simulink model "RaceCar_7DOF_ActiveSuspension"  (R2026a)
settings: Solver=ode4  StopTime=5  FixedStep=0.001
undefined symbols (not defined in the file): a, active_mode, b, bump_duration, bump_height, c_sf, C_sky, c_sr, controller_mode, F_act_max, Ixx, Iyy, K_lqr, k_sf, k_sr, k_t, kerb_duration, kerb_height, m_s, m_uf, m_ur, phi0, phi_dot0, sweep_amplitude, sweep_time, t_bump_front, t_bump_rear, t_f, t_kerb_front, t_kerb_rear, t_r, theta0, theta_dot0, z_s0, z_s_dot0, z_u_FL0, z_u_FL_dot0, z_u_FR0, z_u_FR_dot0, z_u_RL0, z_u_RL_dot0, z_u_RR0, z_u_RR_dot0
libraries: simulink x1
settings Model: Creator=chami  LastModifiedBy=chami

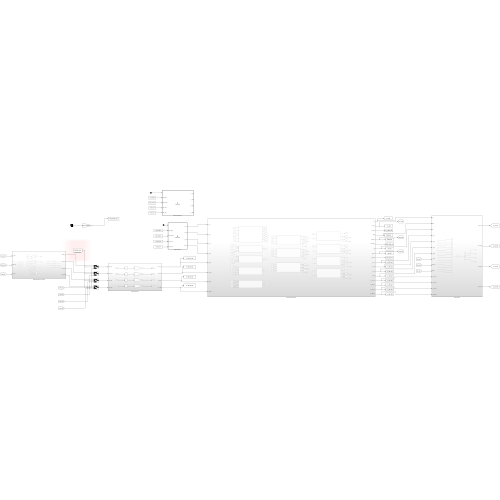
[thumbnail: Simulink's stored preview of the top-level diagram]
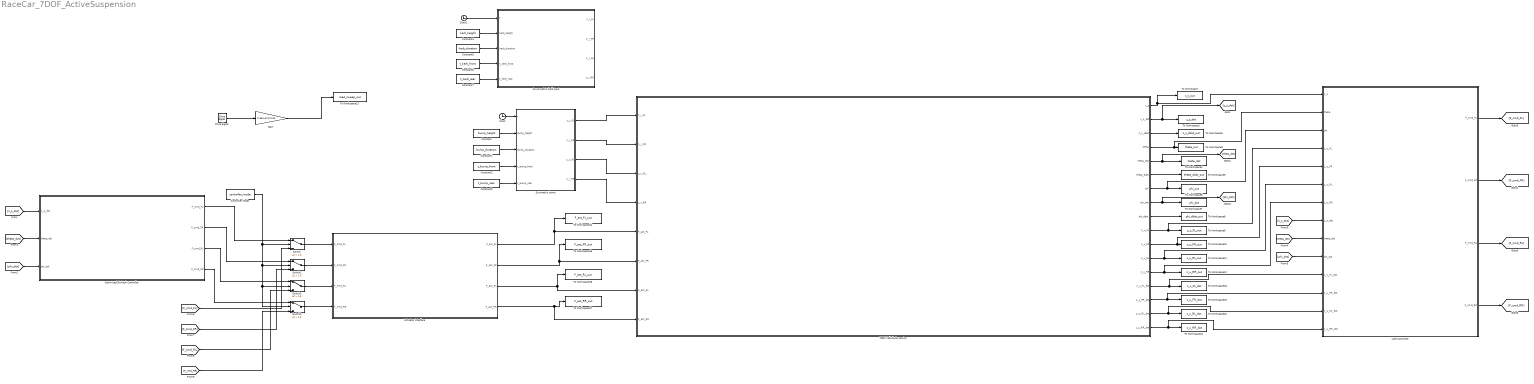
== system RaceCar_7DOF_ActiveSuspension ==
  7DOF Vehicle Dynamics : Subsystem
  Actuator Interface : Subsystem
  Asymmetric Kerb Input : MATLAB Function  TreatAsAtomicUnit=on
  Chirp Signal : simulink/Sources/Chirp Signal  f1=sweep_f_start  T=sweep_time  f2=sweep_f_end
  Clock : Clock
  Clock1 : Clock
  Constant : Constant  Value=bump_height
  Constant1 : Constant  Value=bump_duration
  Constant2 : Constant  Value=t_bump_front
  Constant3 : Constant  Value=t_bump_rear
  Constant4 : Constant  Value=kerb_height
  Constant5 : Constant  Value=kerb_duration
  Constant6 : Constant  Value=t_kerb_front
  Constant7 : Constant  Value=t_kerb_rear
  Controller Mode : Constant  Value=controller_mode
  Gain : Gain  Gain=sweep_amplitude
  LQR Controller : Subsystem
  Optimized Skyhook Controller : Subsystem
  Switch{,1..3} (4 alike) : Switch  Criteria=u2 > Threshold  Threshold=1.5  SaturateOnIntegerOverflow=off  InputSameDT=off
  Symmetric bump : MATLAB Function  TreatAsAtomicUnit=on
  To Workspace : ToWorkspace  VariableName=z_s_out  SaveFormat=Timeseries  SampleTime=-1
  To Workspace1 : ToWorkspace  VariableName=z_s_dot  SaveFormat=Timeseries  SampleTime=-1
  To Workspace10 : ToWorkspace  VariableName=z_u_FR_out  SaveFormat=Timeseries  SampleTime=-1
  To Workspace11 : ToWorkspace  VariableName=z_u_RL_out  SaveFormat=Timeseries  SampleTime=-1
  To Workspace12 : ToWorkspace  VariableName=z_u_RR_out  SaveFormat=Timeseries  SampleTime=-1
  To Workspace13 : ToWorkspace  VariableName=road_sweep_out  SaveFormat=Timeseries  SampleTime=-1
  To Workspace14 : ToWorkspace  VariableName=F_act_FL_out  SaveFormat=Timeseries  SampleTime=-1
  To Workspace15 : ToWorkspace  VariableName=F_act_FR_out  SaveFormat=Timeseries  SampleTime=-1
  To Workspace16 : ToWorkspace  VariableName=F_act_RL_out  SaveFormat=Timeseries  SampleTime=-1
  To Workspace17 : ToWorkspace  VariableName=F_act_RR_out  SaveFormat=Timeseries  SampleTime=-1
  To Workspace18 : ToWorkspace  VariableName=z_u_FL_dot  SaveFormat=Timeseries  SampleTime=-1
  To Workspace19 : ToWorkspace  VariableName=z_u_FR_dot  SaveFormat=Timeseries  SampleTime=-1
  To Workspace2 : ToWorkspace  VariableName=z_s_ddot_out  SaveFormat=Timeseries  SampleTime=-1
  To Workspace20 : ToWorkspace  VariableName=z_u_RL_dot  SaveFormat=Timeseries  SampleTime=-1
  To Workspace21 : ToWorkspace  VariableName=z_u_RR_dot  SaveFormat=Timeseries  SampleTime=-1
  To Workspace3 : ToWorkspace  VariableName=theta_out  SaveFormat=Timeseries  SampleTime=-1
  To Workspace4 : ToWorkspace  VariableName=theta_dot  SaveFormat=Timeseries  SampleTime=-1
  To Workspace5 : ToWorkspace  VariableName=theta_ddot_out  SaveFormat=Timeseries  SampleTime=-1
  To Workspace6 : ToWorkspace  VariableName=phi_out  SaveFormat=Timeseries  SampleTime=-1
  To Workspace7 : ToWorkspace  VariableName=phi_dot  SaveFormat=Timeseries  SampleTime=-1
  To Workspace8 : ToWorkspace  VariableName=phi_ddot_out  SaveFormat=Timeseries  SampleTime=-1
  To Workspace9 : ToWorkspace  VariableName=z_u_FL_out  SaveFormat=Timeseries  SampleTime=-1
  wires:
  7DOF Vehicle Dynamics/1(z_s) -> To Workspace/1, LQR Controller/1(z_s)
  7DOF Vehicle Dynamics/2(z_s_dot) -> [z_s_dot], To Workspace1/1
  7DOF Vehicle Dynamics/3(z_s_ddot) -> To Workspace2/1
  7DOF Vehicle Dynamics/6(theta_ddot) -> To Workspace5/1
  7DOF Vehicle Dynamics/5(theta_dot) -> To Workspace4/1, [theta_dot]
  7DOF Vehicle Dynamics/4(theta) -> LQR Controller/2(theta), To Workspace3/1
  7DOF Vehicle Dynamics/8(phi_dot) -> [phi_dot], To Workspace7/1
  7DOF Vehicle Dynamics/7(phi) -> LQR Controller/3(phi), To Workspace6/1
  7DOF Vehicle Dynamics/9(phi_ddot) -> To Workspace8/1
  7DOF Vehicle Dynamics/10(z_u_FL) -> LQR Controller/4(z_u_FL), To Workspace9/1
  7DOF Vehicle Dynamics/11(z_u_FR) -> LQR Controller/5(z_u_FR), To Workspace10/1
  7DOF Vehicle Dynamics/12(z_u_RL) -> LQR Controller/6(z_u_RL), To Workspace11/1
  7DOF Vehicle Dynamics/13(z_u_RR) -> LQR Controller/7(z_u_RR), To Workspace12/1
  Clock/1 -> Symmetric bump/1(t)
  Constant/1 -> Symmetric bump/2(bump_height)
  Constant1/1 -> Symmetric bump/3(bump_duration)
  Constant2/1 -> Symmetric bump/4(t_bump_front)
  Constant3/1 -> Symmetric bump/5(t_bump_rear)
  Chirp Signal/1 -> Gain/1
  Gain/1 -> To Workspace13/1
  Actuator Interface/1(F_act_FL) -> To Workspace14/1, 7DOF Vehicle Dynamics/5(F_act_FL)
  Actuator Interface/2(F_act_FR) -> To Workspace15/1, 7DOF Vehicle Dynamics/6(F_act_FR)
  Actuator Interface/3(F_act_RL) -> To Workspace16/1, 7DOF Vehicle Dynamics/7(F_act_RL)
  Actuator Interface/4(F_act_RR) -> To Workspace17/1, 7DOF Vehicle Dynamics/8(F_act_RR)
  [z_s_dot] -> Optimized Skyhook Controller/1(z_s_dot)
  [theta_dot] -> Optimized Skyhook Controller/2(theta_dot)
  [phi_dot] -> Optimized Skyhook Controller/3(phi_dot)
  Clock1/1 -> Asymmetric Kerb Input/1(t)
  Constant4/1 -> Asymmetric Kerb Input/2(kerb_height)
  Constant5/1 -> Asymmetric Kerb Input/3(kerb_duration)
  Constant6/1 -> Asymmetric Kerb Input/4(t_kerb_front)
  Constant7/1 -> Asymmetric Kerb Input/5(t_kerb_rear)
  7DOF Vehicle Dynamics/14(z_u_FL_dot) -> LQR Controller/11(z_u_FL_dot), To Workspace18/1
  7DOF Vehicle Dynamics/15(z_u_FR_dot) -> LQR Controller/12(z_u_FR_dot), To Workspace19/1
  7DOF Vehicle Dynamics/16(z_u_RL_dot) -> LQR Controller/13(z_u_RL_dot), To Workspace20/1
  7DOF Vehicle Dynamics/17(z_u_RR_dot) -> LQR Controller/14(z_u_RR_dot), To Workspace21/1
  [phi_dot] -> LQR Controller/10(phi_dot)
  [theta_dot] -> LQR Controller/9(theta_dot)
  [z_s_dot] -> LQR Controller/8(z_s_dot)
  LQR Controller/1(F_cmd_FL) -> [F_cmd_FL]
  LQR Controller/2(F_cmd_FR) -> [F_cmd_FR]
  LQR Controller/3(F_cmd_RL) -> [F_cmd_RL]
  LQR Controller/4(F_cmd_RR) -> [F_cmd_RR]
  Symmetric bump/1(z_r_FL) -> 7DOF Vehicle Dynamics/1(z_r_FL)
  Symmetric bump/2(z_r_FR) -> 7DOF Vehicle Dynamics/2(z_r_FR)
  Symmetric bump/3(z_r_RL) -> 7DOF Vehicle Dynamics/3(z_r_RL)
  Symmetric bump/4(z_r_RR) -> 7DOF Vehicle Dynamics/4(z_r_RR)
  Switch/1 -> Actuator Interface/1("F_cmd_FL ")
  Switch1/1 -> Actuator Interface/2(F_cmd_FR)
  Switch2/1 -> Actuator Interface/3(F_cmd_RL)
  Switch3/1 -> Actuator Interface/4(F_cmd_RR)
  Optimized Skyhook Controller/1(F_cmd_FL) -> Switch/1
  Optimized Skyhook Controller/2(F_cmd_FR) -> Switch1/1
  Optimized Skyhook Controller/3(F_cmd_RL) -> Switch2/1
  Optimized Skyhook Controller/4(F_cmd_RR) -> Switch3/1
  [F_cmd_FL] -> Switch/3
  [F_cmd_FR] -> Switch1/3
  [F_cmd_RL] -> Switch2/3
  [F_cmd_RR] -> Switch3/3
  Controller Mode/1 -> Switch/2, Switch1/2, Switch2/2, Switch3/2

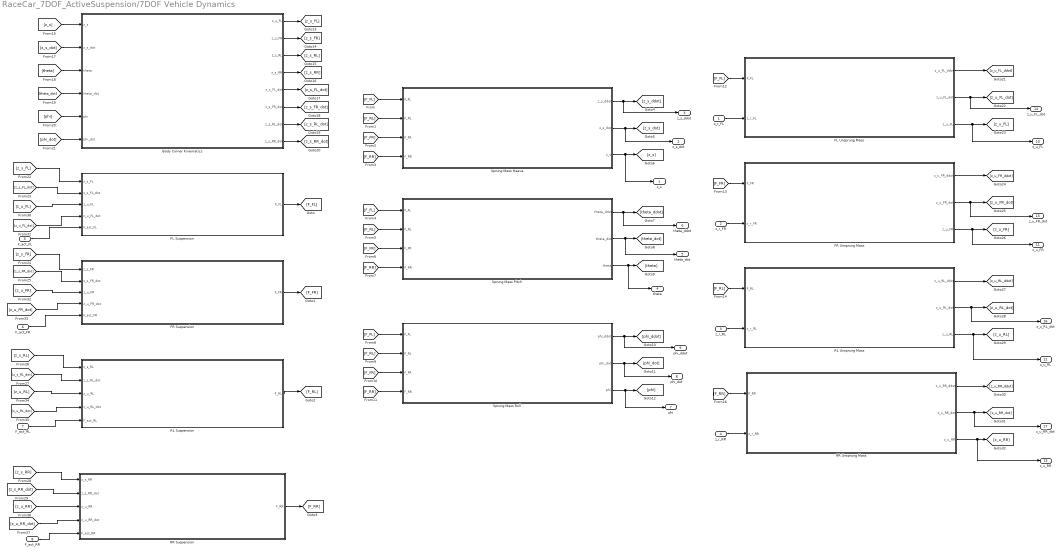
== system RaceCar_7DOF_ActiveSuspension/7DOF Vehicle Dynamics ==
  z_r_FL : Inport
  z_r_FR : Inport  Port=2
  z_r_RL : Inport  Port=3
  z_r_RR : Inport  Port=4
  F_act_FL : Inport  Port=5
  F_act_FR : Inport  Port=6
  F_act_RL : Inport  Port=7
  F_act_RR : Inport  Port=8
  Body Corner Kinematics : Subsystem
  "FL Suspension " : Subsystem
  FL Unsprung Mass : Subsystem
  FR Suspension : Subsystem
  FR Unsprung Mass : Subsystem
  RL Suspension : Subsystem
  RL Unsprung Mass : Subsystem
  RR Suspension : Subsystem
  RR Unsprung Mass : Subsystem
  Sprung Mass Heave : Subsystem
  Sprung Mass Pitch : Subsystem
  Sprung Mass Roll : Subsystem
  z_s : Outport
  z_s_dot : Outport  Port=2
  z_s_ddot : Outport  Port=3
  theta : Outport  Port=4
  theta_dot : Outport  Port=5
  theta_ddot : Outport  Port=6
  phi : Outport  Port=7
  phi_dot : Outport  Port=8
  phi_ddot : Outport  Port=9
  z_u_FL : Outport  Port=10
  z_u_FR : Outport  Port=11
  z_u_RL : Outport  Port=12
  z_u_RR : Outport  Port=13
  z_u_FL_dot : Outport  Port=14
  z_u_FR_dot : Outport  Port=15
  z_u_RL_dot : Outport  Port=16
  z_u_RR_dot : Outport  Port=17
  wires:
  [F_FL] -> Sprung Mass Pitch/1(F_FL)
  Body Corner Kinematics/2(z_s_FR) -> [z_s_FR]
  [z_u_FL_dot] -> "FL Suspension "/4(z_u_FL_dot)
  [phi] -> Body Corner Kinematics/5(phi)
  Sprung Mass Roll/3(phi) -> phi/1, [phi]
  [z_u_RL_dot] -> RL Suspension/4(z_u_RL_dot)
  [F_FR] -> Sprung Mass Roll/3(F_FR)
  [z_s_RL] -> RL Suspension/1(z_s_RL)
  FL Unsprung Mass/2(z_u_FL_dot) -> z_u_FL_dot/1, [z_u_FL_dot]
  [z_s] -> Body Corner Kinematics/1(z_s)
  [theta] -> Body Corner Kinematics/3(theta)
  [z_s_FL] -> "FL Suspension "/1(z_s_FL)
  FR Unsprung Mass/3(z_u_FR) -> z_u_FR/1, [z_u_FR]
  [z_s_RR_dot] -> RR Suspension/2(z_s_RR_dot)
  FL Unsprung Mass/1(z_u_FL_ddot) -> [z_u_FL_ddot]
  Sprung Mass Pitch/1(theta_ddot) -> theta_ddot/1, [theta_ddot]
  Sprung Mass Pitch/3(theta) -> theta/1, [theta]
  [F_RL] -> Sprung Mass Heave/2(F_RL)
  Body Corner Kinematics/1(z_s_FL) -> [z_s_FL]
  [z_s_FR] -> FR Suspension/1(z_s_FR)
  Body Corner Kinematics/4(z_s_RR) -> [z_s_RR]
  [z_u_RR_dot] -> RR Suspension/4(z_u_RR_dot)
  FR Suspension/1(F_FR) -> [F_FR]
  FR Unsprung Mass/1(z_u_FR_ddot) -> [z_u_FR_ddot]
  RL Unsprung Mass/1(z_u_RL_ddot) -> [z_u_RL_ddot]
  [F_FR] -> Sprung Mass Pitch/3(F_FR)
  [F_RL] -> RL Unsprung Mass/1(F_RL)
  Body Corner Kinematics/6(z_s_FR_dot) -> [z_s_FR_dot]
  [z_s_dot] -> Body Corner Kinematics/2(z_s_dot)
  [z_u_FR] -> FR Suspension/3(z_u_FR)
  [z_s_FR_dot] -> FR Suspension/2(z_s_FR_dot)
  RR Suspension/1(F_RR) -> [F_RR]
  Sprung Mass Heave/2(z_s_dot) -> z_s_dot/1, [z_s_dot]
  Sprung Mass Roll/2(phi_dot) -> phi_dot/1, [phi_dot]
  Body Corner Kinematics/5(z_s_FL_dot) -> [z_s_FL_dot]
  [z_u_FL] -> "FL Suspension "/3(z_u_FL)
  [z_u_RL] -> RL Suspension/3(z_u_RL)
  Sprung Mass Heave/1(z_s_ddot) -> z_s_ddot/1, [z_s_ddot]
  [z_s_RR] -> RR Suspension/1(z_s_RR)
  [F_RR] -> Sprung Mass Heave/4(F_RR)
  [F_FL] -> FL Unsprung Mass/1(F_FL)
  [theta_dot] -> Body Corner Kinematics/4(theta_dot)
  [F_FL] -> Sprung Mass Heave/1(F_FL)
  [F_FL] -> Sprung Mass Roll/1(F_FL)
  [z_s_FL_dot] -> "FL Suspension "/2(z_s_FL_dot)
  Body Corner Kinematics/8(z_s_RR_dot) -> [z_s_RR_dot]
  [F_RR] -> RR Unsprung Mass/1(F_RR)
  [z_u_FR_dot] -> FR Suspension/4(z_u_FR_dot)
  [z_u_RR] -> RR Suspension/3(z_u_RR)
  [F_RL] -> Sprung Mass Pitch/2(F_RL)
  Sprung Mass Heave/3(z_s) -> z_s/1, [z_s]
  RL Suspension/1(F_RL) -> [F_RL]
  RR Unsprung Mass/3(z_u_RR) -> z_u_RR/1, [z_u_RR]
  FL Unsprung Mass/3(z_u_FL) -> z_u_FL/1, [z_u_FL]
  RL Unsprung Mass/3(z_u_RL) -> z_u_RL/1, [z_u_RL]
  FR Unsprung Mass/2(z_u_FR_dot) -> z_u_FR_dot/1, [z_u_FR_dot]
  [F_FR] -> FR Unsprung Mass/1(F_FR)
  "FL Suspension "/1(F_FL) -> [F_FL]
  [F_RR] -> Sprung Mass Roll/4(F_RR)
  Sprung Mass Roll/1(phi_ddot) -> phi_ddot/1, [phi_ddot]
  RR Unsprung Mass/1(z_u_RR_ddot) -> [z_u_RR_ddot]
  [F_RR] -> Sprung Mass Pitch/4(F_RR)
  RR Unsprung Mass/2(z_u_RR_dot) -> z_u_RR_dot/1, [z_u_RR_dot]
  [F_RL] -> Sprung Mass Roll/2(F_RL)
  Sprung Mass Pitch/2(theta_dot) -> theta_dot/1, [theta_dot]
  [F_FR] -> Sprung Mass Heave/3(F_FR)
  [z_s_RL_dot] -> RL Suspension/2(z_s_RL_dot)
  [phi_dot] -> Body Corner Kinematics/6(phi_dot)
  Body Corner Kinematics/7(z_s_RL_dot) -> [z_s_RL_dot]
  RL Unsprung Mass/2(z_u_RL_dot) -> z_u_RL_dot/1, [z_u_RL_dot]
  Body Corner Kinematics/3(z_s_RL) -> [z_s_RL]
  z_r_FL/1 -> FL Unsprung Mass/2(z_r_FL)
  z_r_FR/1 -> FR Unsprung Mass/2(z_r_FR)
  z_r_RL/1 -> RL Unsprung Mass/2(z_r_RL)
  z_r_RR/1 -> RR Unsprung Mass/2(z_r_RR)
  F_act_FL/1 -> "FL Suspension "/5(F_act_FL)
  F_act_FR/1 -> FR Suspension/5(F_act_FR)
  F_act_RL/1 -> RL Suspension/5(F_act_RL)
  F_act_RR/1 -> RR Suspension/5(F_act_RR)

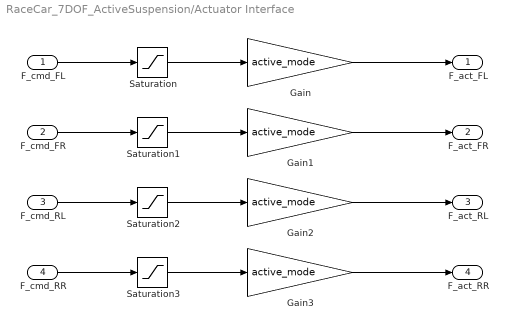
== system RaceCar_7DOF_ActiveSuspension/Actuator Interface ==
  "F_cmd_FL " : Inport
  F_cmd_FR : Inport  Port=2
  F_cmd_RL : Inport  Port=3
  F_cmd_RR : Inport  Port=4
  Gain{,1..3} (4 alike) : Gain  Gain=active_mode
  Saturation{,1..3} (4 alike) : Saturate  UpperLimit=F_act_max  LowerLimit=-F_act_max
  F_act_FL : Outport
  F_act_FR : Outport  Port=2
  F_act_RL : Outport  Port=3
  F_act_RR : Outport  Port=4
  wires:
  Saturation/1 -> Gain/1
  Saturation1/1 -> Gain1/1
  Saturation2/1 -> Gain2/1
  Saturation3/1 -> Gain3/1
  "F_cmd_FL "/1 -> Saturation/1
  F_cmd_FR/1 -> Saturation1/1
  F_cmd_RL/1 -> Saturation2/1
  F_cmd_RR/1 -> Saturation3/1
  Gain/1 -> F_act_FL/1
  Gain1/1 -> F_act_FR/1
  Gain2/1 -> F_act_RL/1
  Gain3/1 -> F_act_RR/1

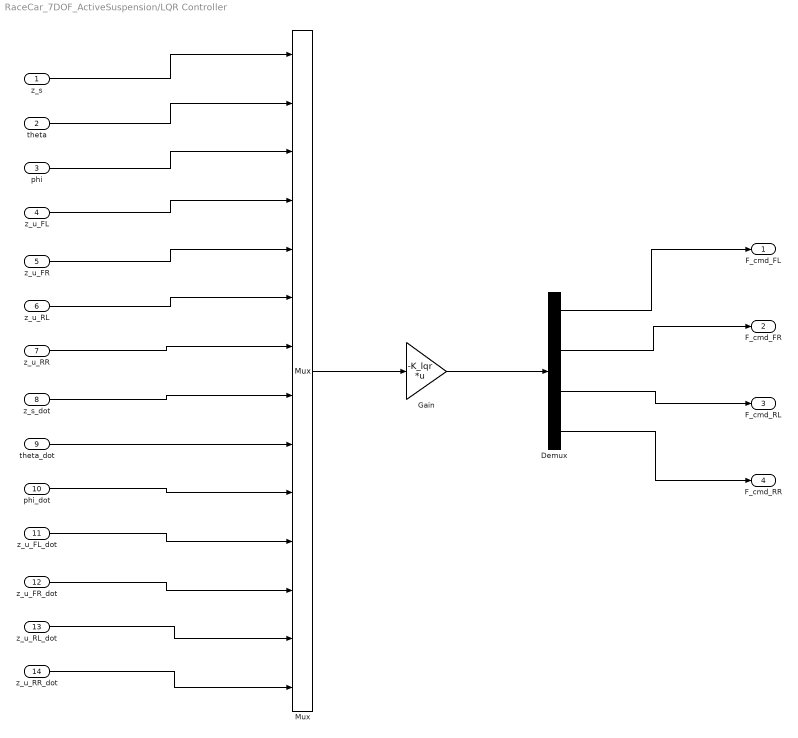
== system RaceCar_7DOF_ActiveSuspension/LQR Controller ==
  z_s : Inport
  theta : Inport  Port=2
  phi : Inport  Port=3
  z_u_FL : Inport  Port=4
  z_u_FR : Inport  Port=5
  z_u_RL : Inport  Port=6
  z_u_RR : Inport  Port=7
  z_s_dot : Inport  Port=8
  theta_dot : Inport  Port=9
  phi_dot : Inport  Port=10
  z_u_FL_dot : Inport  Port=11
  z_u_FR_dot : Inport  Port=12
  z_u_RL_dot : Inport  Port=13
  z_u_RR_dot : Inport  Port=14
  Demux : Demux
  Gain : Gain  Gain=-K_lqr  Multiplication=Matrix(K*u)
  Mux : Mux  Inputs=14
  F_cmd_FL : Outport
  F_cmd_FR : Outport  Port=2
  F_cmd_RL : Outport  Port=3
  F_cmd_RR : Outport  Port=4
  wires:
  z_s/1 -> Mux/1
  theta/1 -> Mux/2
  phi/1 -> Mux/3
  z_u_FL/1 -> Mux/4
  z_u_FR/1 -> Mux/5
  z_u_RL/1 -> Mux/6
  z_u_RR/1 -> Mux/7
  z_s_dot/1 -> Mux/8
  theta_dot/1 -> Mux/9
  phi_dot/1 -> Mux/10
  z_u_FL_dot/1 -> Mux/11
  z_u_FR_dot/1 -> Mux/12
  z_u_RL_dot/1 -> Mux/13
  z_u_RR_dot/1 -> Mux/14
  Mux/1 -> Gain/1
  Gain/1 -> Demux/1
  Demux/1 -> F_cmd_FL/1
  Demux/2 -> F_cmd_FR/1
  Demux/3 -> F_cmd_RL/1
  Demux/4 -> F_cmd_RR/1

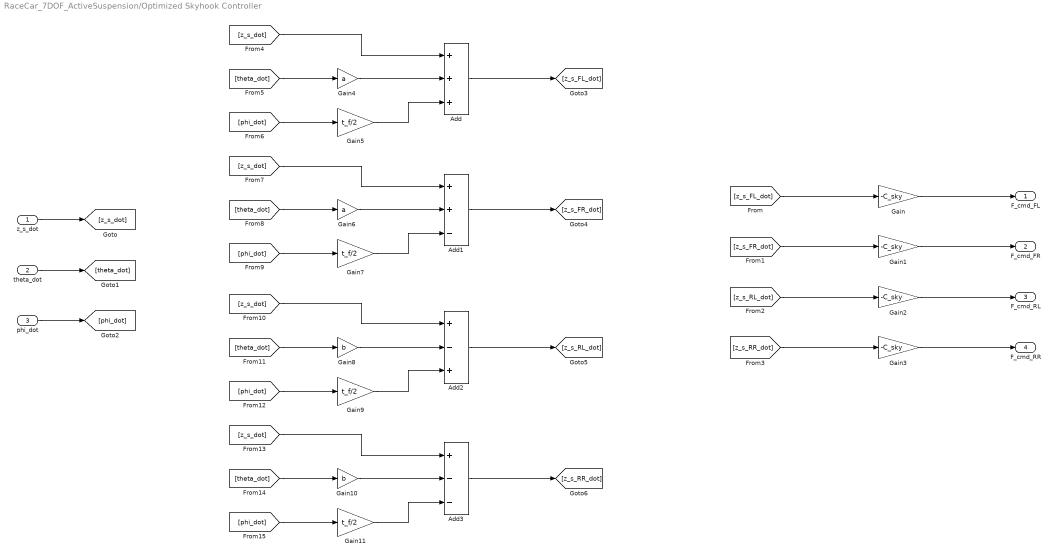
== system RaceCar_7DOF_ActiveSuspension/Optimized Skyhook Controller ==
  z_s_dot : Inport
  theta_dot : Inport  Port=2
  phi_dot : Inport  Port=3
  Add : Sum  Inputs=+++
  Add1 : Sum  Inputs=++-
  Add2 : Sum  Inputs=+-+
  Add3 : Sum  Inputs=+--
  Gain{,1..3} (4 alike) : Gain  Gain=-C_sky
  Gain10 : Gain  Gain=b
  Gain{5,7,9,11} (4 alike) : Gain  Gain=t_f/2
  Gain4 : Gain  Gain=a
  Gain6 : Gain  Gain=a
  Gain8 : Gain  Gain=b
  F_cmd_FL : Outport
  F_cmd_FR : Outport  Port=2
  F_cmd_RL : Outport  Port=3
  F_cmd_RR : Outport  Port=4
  wires:
  [z_s_FL_dot] -> Gain/1
  [z_s_FR_dot] -> Gain1/1
  [z_s_RL_dot] -> Gain2/1
  [z_s_RR_dot] -> Gain3/1
  Gain/1 -> F_cmd_FL/1
  Gain1/1 -> F_cmd_FR/1
  Gain2/1 -> F_cmd_RL/1
  Gain3/1 -> F_cmd_RR/1
  z_s_dot/1 -> [z_s_dot]
  theta_dot/1 -> [theta_dot]
  phi_dot/1 -> [phi_dot]
  [theta_dot] -> Gain4/1
  [phi_dot] -> Gain5/1
  Gain4/1 -> Add/2
  [z_s_dot] -> Add/1
  Gain5/1 -> Add/3
  Add/1 -> [z_s_FL_dot]
  Add1/1 -> [z_s_FR_dot]
  Gain7/1 -> Add1/3
  [z_s_dot] -> Add1/1
  Gain6/1 -> Add1/2
  [phi_dot] -> Gain7/1
  [theta_dot] -> Gain6/1
  [theta_dot] -> Gain10/1
  [phi_dot] -> Gain11/1
  Gain10/1 -> Add3/2
  [z_s_dot] -> Add3/1
  Gain11/1 -> Add3/3
  Add3/1 -> [z_s_RR_dot]
  Add2/1 -> [z_s_RL_dot]
  Gain9/1 -> Add2/3
  [z_s_dot] -> Add2/1
  Gain8/1 -> Add2/2
  [phi_dot] -> Gain9/1
  [theta_dot] -> Gain8/1

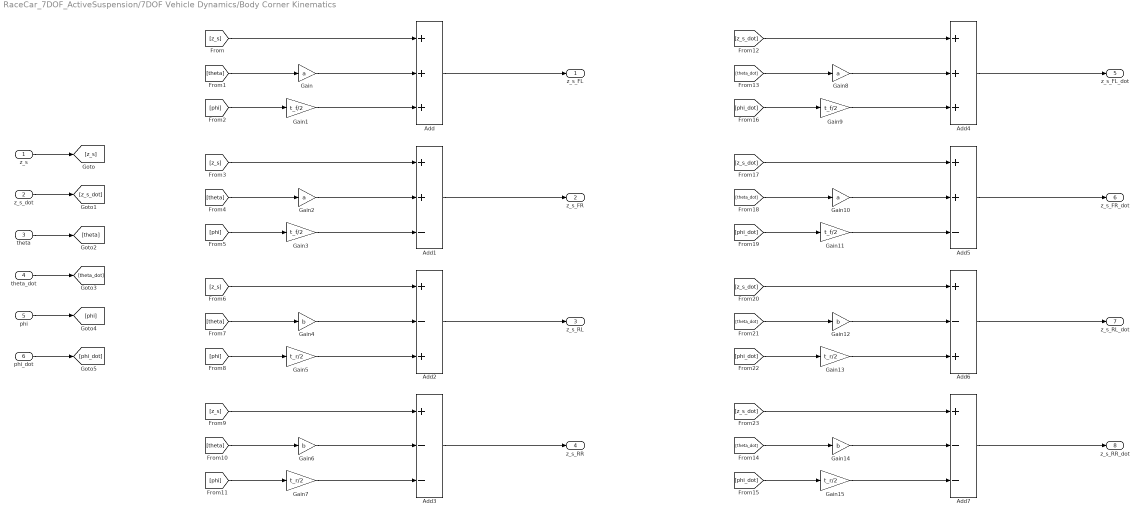
== system RaceCar_7DOF_ActiveSuspension/7DOF Vehicle Dynamics/Body Corner Kinematics ==
  z_s : Inport
  z_s_dot : Inport  Port=2
  theta : Inport  Port=3
  theta_dot : Inport  Port=4
  phi : Inport  Port=5
  phi_dot : Inport  Port=6
  Add : Sum  Inputs=+++
  Add1 : Sum  Inputs=++-
  Add2 : Sum  Inputs=+-+
  Add3 : Sum  Inputs=+--
  Add4 : Sum  Inputs=+++
  Add5 : Sum  Inputs=++-
  Add6 : Sum  Inputs=+-+
  Add7 : Sum  Inputs=+--
  Gain{,2,8,10} (4 alike) : Gain  Gain=a
  Gain{1,3,9,11} (4 alike) : Gain  Gain=t_f/2
  Gain{4,6,12,14} (4 alike) : Gain  Gain=b
  Gain{5,7,13,15} (4 alike) : Gain  Gain=t_r/2
  z_s_FL : Outport
  z_s_FR : Outport  Port=2
  z_s_RL : Outport  Port=3
  z_s_RR : Outport  Port=4
  z_s_FL_dot : Outport  Port=5
  z_s_FR_dot : Outport  Port=6
  z_s_RL_dot : Outport  Port=7
  z_s_RR_dot : Outport  Port=8
  wires:
  Gain/1 -> Add/2
  Gain1/1 -> Add/3
  Add/1 -> z_s_FL/1
  z_s/1 -> [z_s]
  z_s_dot/1 -> [z_s_dot]
  theta/1 -> [theta]
  theta_dot/1 -> [theta_dot]
  phi/1 -> [phi]
  phi_dot/1 -> [phi_dot]
  [z_s] -> Add/1
  [theta] -> Gain/1
  [phi] -> Gain1/1
  [phi] -> Gain3/1
  [theta] -> Gain2/1
  [z_s] -> Add1/1
  Add1/1 -> z_s_FR/1
  Gain3/1 -> Add1/3
  Gain2/1 -> Add1/2
  [phi] -> Gain5/1
  [theta] -> Gain4/1
  [z_s] -> Add2/1
  Add2/1 -> z_s_RL/1
  Gain5/1 -> Add2/3
  Gain4/1 -> Add2/2
  Gain6/1 -> Add3/2
  Gain7/1 -> Add3/3
  Add3/1 -> z_s_RR/1
  [z_s] -> Add3/1
  [theta] -> Gain6/1
  [phi] -> Gain7/1
  [phi_dot] -> Gain15/1
  [theta_dot] -> Gain14/1
  [z_s_dot] -> Add7/1
  Add7/1 -> z_s_RR_dot/1
  Gain15/1 -> Add7/3
  Gain14/1 -> Add7/2
  Gain12/1 -> Add6/2
  Gain13/1 -> Add6/3
  Add6/1 -> z_s_RL_dot/1
  [z_s_dot] -> Add6/1
  [theta_dot] -> Gain12/1
  [phi_dot] -> Gain13/1
  Gain10/1 -> Add5/2
  Gain11/1 -> Add5/3
  Add5/1 -> z_s_FR_dot/1
  [z_s_dot] -> Add5/1
  [theta_dot] -> Gain10/1
  [phi_dot] -> Gain11/1
  [phi_dot] -> Gain9/1
  [theta_dot] -> Gain8/1
  [z_s_dot] -> Add4/1
  Add4/1 -> z_s_FL_dot/1
  Gain9/1 -> Add4/3
  Gain8/1 -> Add4/2

== system RaceCar_7DOF_ActiveSuspension/7DOF Vehicle Dynamics/FL Suspension  ==
  z_s_FL : Inport
  z_s_FL_dot : Inport  Port=2
  z_u_FL : Inport  Port=3
  z_u_FL_dot : Inport  Port=4
  F_act_FL : Inport  Port=5
  Add : Sum  Inputs=+-
  Add1 : Sum  Inputs=+-
  Add2 : Sum  Inputs=+++
  Gain : Gain  Gain=-k_sf
  Gain1 : Gain  Gain=-c_sf
  F_FL : Outport
  wires:
  z_u_FL/1 -> Add/2
  z_s_FL/1 -> Add/1
  z_u_FL_dot/1 -> Add1/2
  z_s_FL_dot/1 -> Add1/1
  Add/1 -> Gain/1  "delta_FL"
  Add1/1 -> Gain1/1  "delta_FL_dot"
  Add2/1 -> F_FL/1
  Gain/1 -> Add2/1  "Fs_FL"
  Gain1/1 -> Add2/2  "Fd_FL"
  F_act_FL/1 -> Add2/3

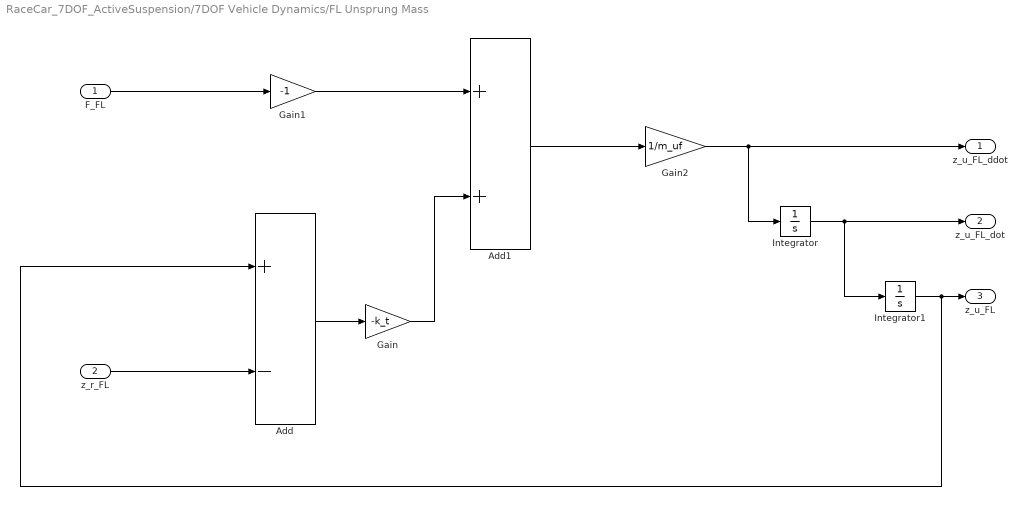
== system RaceCar_7DOF_ActiveSuspension/7DOF Vehicle Dynamics/FL Unsprung Mass ==
  F_FL : Inport
  z_r_FL : Inport  Port=2
  Add : Sum  Inputs=+-
  Add1 : Sum
  Gain : Gain  Gain=-k_t
  Gain1 : Gain  Gain=-1
  Gain2 : Gain  Gain=1/m_uf
  Integrator : Integrator  InitialCondition=z_u_FL_dot0
  Integrator1 : Integrator  InitialCondition=z_u_FL0
  z_u_FL_ddot : Outport
  z_u_FL_dot : Outport  Port=2
  z_u_FL : Outport  Port=3
  wires:
  Integrator1/1 -> Add/1, z_u_FL/1
  Integrator/1 -> z_u_FL_dot/1, Integrator1/1
  z_r_FL/1 -> Add/2
  Add/1 -> Gain/1
  Gain/1 -> Add1/2
  F_FL/1 -> Gain1/1
  Gain1/1 -> Add1/1
  Add1/1 -> Gain2/1
  Gain2/1 -> Integrator/1, z_u_FL_ddot/1

== system RaceCar_7DOF_ActiveSuspension/7DOF Vehicle Dynamics/FR Suspension ==
  z_s_FR : Inport
  z_s_FR_dot : Inport  Port=2
  z_u_FR : Inport  Port=3
  z_u_FR_dot : Inport  Port=4
  F_act_FR : Inport  Port=5
  Add : Sum  Inputs=+-
  Add1 : Sum  Inputs=+-
  Add2 : Sum  Inputs=+++
  Gain : Gain  Gain=-k_sf
  Gain1 : Gain  Gain=-c_sf
  F_FR : Outport
  wires:
  Gain1/1 -> Add2/2  "Fd_FR"
  Gain/1 -> Add2/1  "Fs_FR"
  Add2/1 -> F_FR/1
  Add1/1 -> Gain1/1  "delta_FR_dot"
  Add/1 -> Gain/1  "delta_FR"
  z_s_FR_dot/1 -> Add1/1
  z_u_FR_dot/1 -> Add1/2
  z_s_FR/1 -> Add/1
  z_u_FR/1 -> Add/2
  F_act_FR/1 -> Add2/3

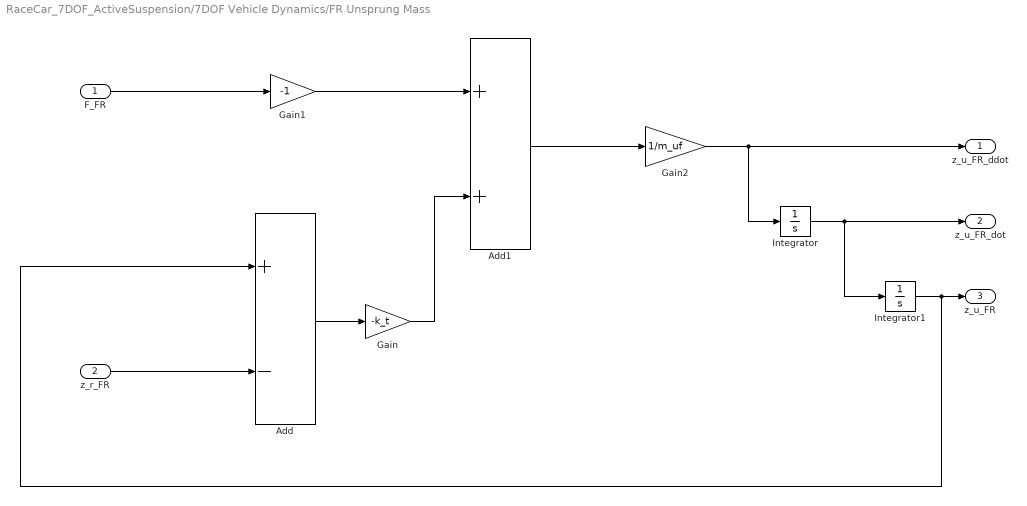
== system RaceCar_7DOF_ActiveSuspension/7DOF Vehicle Dynamics/FR Unsprung Mass ==
  F_FR : Inport
  z_r_FR : Inport  Port=2
  Add : Sum  Inputs=+-
  Add1 : Sum
  Gain : Gain  Gain=-k_t
  Gain1 : Gain  Gain=-1
  Gain2 : Gain  Gain=1/m_uf
  Integrator : Integrator  InitialCondition=z_u_FR_dot0
  Integrator1 : Integrator  InitialCondition=z_u_FR0
  z_u_FR_ddot : Outport
  z_u_FR_dot : Outport  Port=2
  z_u_FR : Outport  Port=3
  wires:
  Gain2/1 -> z_u_FR_ddot/1, Integrator/1
  Add1/1 -> Gain2/1
  Gain1/1 -> Add1/1
  F_FR/1 -> Gain1/1
  Gain/1 -> Add1/2
  Add/1 -> Gain/1
  z_r_FR/1 -> Add/2
  Integrator/1 -> Integrator1/1, z_u_FR_dot/1
  Integrator1/1 -> z_u_FR/1, Add/1

== system RaceCar_7DOF_ActiveSuspension/7DOF Vehicle Dynamics/RL Suspension ==
  z_s_RL : Inport
  z_s_RL_dot : Inport  Port=2
  z_u_RL : Inport  Port=3
  z_u_RL_dot : Inport  Port=4
  F_act_RL : Inport  Port=5
  Add : Sum  Inputs=+-
  Add1 : Sum  Inputs=+-
  Add2 : Sum  Inputs=+++
  Gain : Gain  Gain=-k_sr
  Gain1 : Gain  Gain=-c_sr
  F_RL : Outport
  wires:
  Gain1/1 -> Add2/2  "Fd_RL"
  Gain/1 -> Add2/1  "Fs_RL"
  Add2/1 -> F_RL/1
  Add1/1 -> Gain1/1  "delta_RL_dot"
  Add/1 -> Gain/1  "delta_RL"
  z_s_RL_dot/1 -> Add1/1
  z_u_RL_dot/1 -> Add1/2
  z_s_RL/1 -> Add/1
  z_u_RL/1 -> Add/2
  F_act_RL/1 -> Add2/3

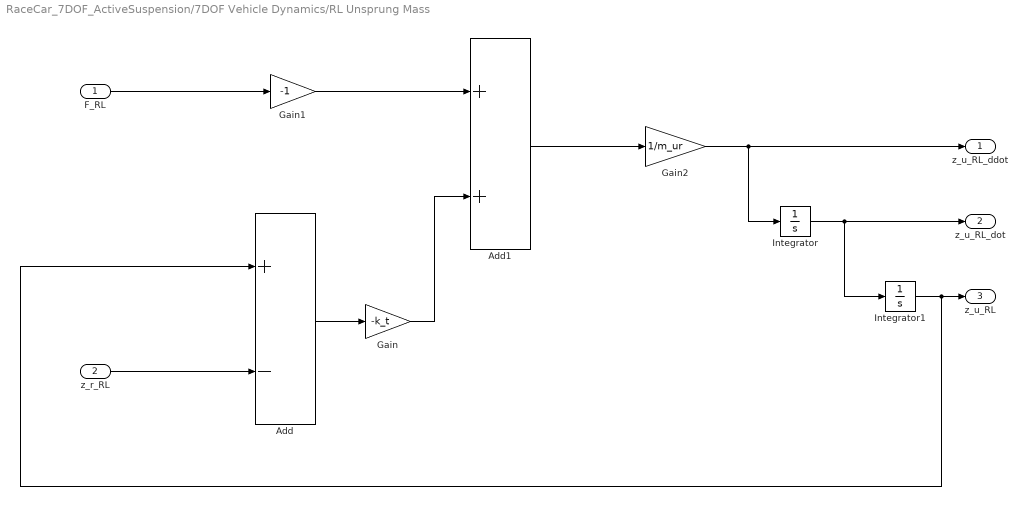
== system RaceCar_7DOF_ActiveSuspension/7DOF Vehicle Dynamics/RL Unsprung Mass ==
  F_RL : Inport
  z_r_RL : Inport  Port=2
  Add : Sum  Inputs=+-
  Add1 : Sum
  Gain : Gain  Gain=-k_t
  Gain1 : Gain  Gain=-1
  Gain2 : Gain  Gain=1/m_ur
  Integrator : Integrator  InitialCondition=z_u_RL_dot0
  Integrator1 : Integrator  InitialCondition=z_u_RL0
  z_u_RL_ddot : Outport
  z_u_RL_dot : Outport  Port=2
  z_u_RL : Outport  Port=3
  wires:
  Gain2/1 -> z_u_RL_ddot/1, Integrator/1
  Add1/1 -> Gain2/1
  Gain1/1 -> Add1/1
  F_RL/1 -> Gain1/1
  Gain/1 -> Add1/2
  Add/1 -> Gain/1
  z_r_RL/1 -> Add/2
  Integrator/1 -> Integrator1/1, z_u_RL_dot/1
  Integrator1/1 -> z_u_RL/1, Add/1

== system RaceCar_7DOF_ActiveSuspension/7DOF Vehicle Dynamics/RR Suspension ==
  z_s_RR : Inport
  z_s_RR_dot : Inport  Port=2
  z_u_RR : Inport  Port=3
  z_u_RR_dot : Inport  Port=4
  F_act_RR : Inport  Port=5
  Add : Sum  Inputs=+-
  Add1 : Sum  Inputs=+-
  Add2 : Sum  Inputs=+++
  Gain : Gain  Gain=-k_sr
  Gain1 : Gain  Gain=-c_sr
  F_RR : Outport
  wires:
  z_u_RR/1 -> Add/2
  z_s_RR/1 -> Add/1
  z_u_RR_dot/1 -> Add1/2
  z_s_RR_dot/1 -> Add1/1
  Add/1 -> Gain/1  "delta_RR"
  Add1/1 -> Gain1/1  "delta_RR_dot"
  Add2/1 -> F_RR/1
  Gain/1 -> Add2/1  "Fs_RR"
  Gain1/1 -> Add2/2  "Fd_RR"
  F_act_RR/1 -> Add2/3

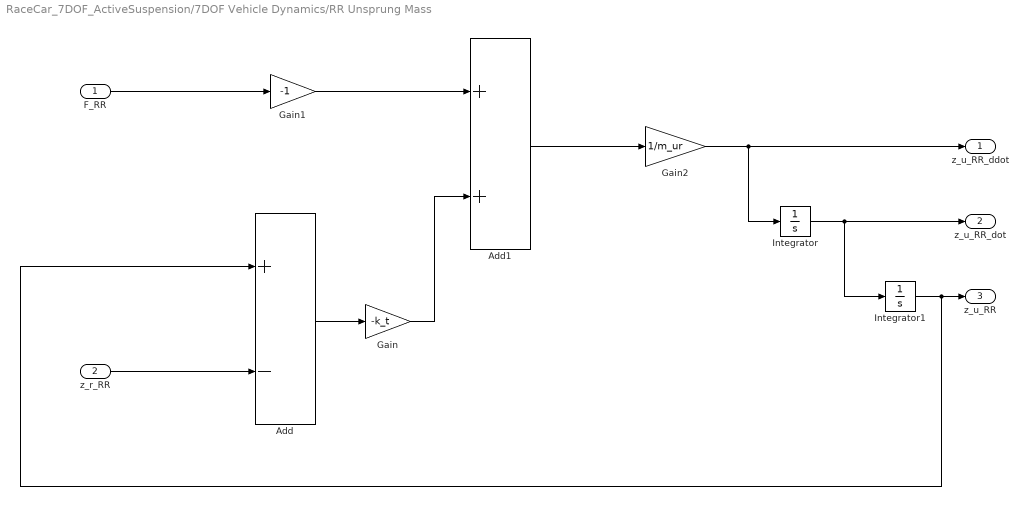
== system RaceCar_7DOF_ActiveSuspension/7DOF Vehicle Dynamics/RR Unsprung Mass ==
  F_RR : Inport
  z_r_RR : Inport  Port=2
  Add : Sum  Inputs=+-
  Add1 : Sum
  Gain : Gain  Gain=-k_t
  Gain1 : Gain  Gain=-1
  Gain2 : Gain  Gain=1/m_ur
  Integrator : Integrator  InitialCondition=z_u_RR_dot0
  Integrator1 : Integrator  InitialCondition=z_u_RR0
  z_u_RR_ddot : Outport
  z_u_RR_dot : Outport  Port=2
  z_u_RR : Outport  Port=3
  wires:
  Integrator1/1 -> Add/1, z_u_RR/1
  Integrator/1 -> z_u_RR_dot/1, Integrator1/1
  z_r_RR/1 -> Add/2
  Add/1 -> Gain/1
  Gain/1 -> Add1/2
  F_RR/1 -> Gain1/1
  Gain1/1 -> Add1/1
  Add1/1 -> Gain2/1
  Gain2/1 -> Integrator/1, z_u_RR_ddot/1

== system RaceCar_7DOF_ActiveSuspension/7DOF Vehicle Dynamics/Sprung Mass Heave ==
  F_FL : Inport
  F_RL : Inport  Port=2
  F_FR : Inport  Port=3
  F_RR : Inport  Port=4
  Add : Sum  Inputs=++++
  Gain : Gain  Gain=1/m_s
  Integrator : Integrator  InitialCondition=z_s_dot0
  Integrator1 : Integrator  InitialCondition=z_s0
  z_s_ddot : Outport
  z_s_dot : Outport  Port=2
  z_s : Outport  Port=3
  wires:
  Add/1 -> Gain/1
  F_RL/1 -> Add/3
  F_RR/1 -> Add/4
  F_FL/1 -> Add/1
  F_FR/1 -> Add/2
  Gain/1 -> Integrator/1, z_s_ddot/1
  Integrator/1 -> Integrator1/1, z_s_dot/1
  Integrator1/1 -> z_s/1

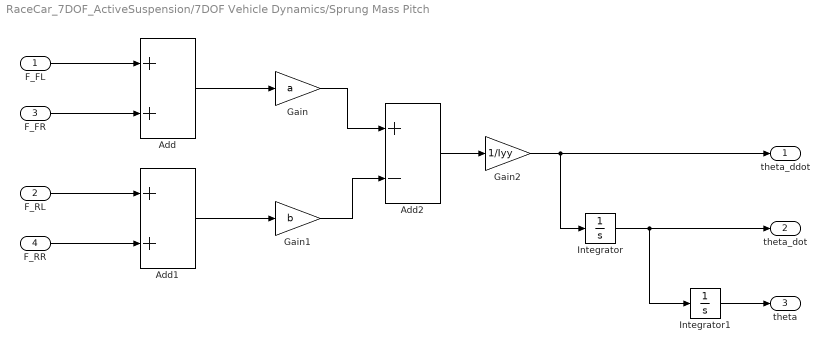
== system RaceCar_7DOF_ActiveSuspension/7DOF Vehicle Dynamics/Sprung Mass Pitch ==
  F_FL : Inport
  F_RL : Inport  Port=2
  F_FR : Inport  Port=3
  F_RR : Inport  Port=4
  Add : Sum
  Add1 : Sum
  Add2 : Sum  Inputs=+-
  Gain : Gain  Gain=a
  Gain1 : Gain  Gain=b
  Gain2 : Gain  Gain=1/Iyy
  Integrator : Integrator  InitialCondition=theta_dot0
  Integrator1 : Integrator  InitialCondition=theta0
  theta_ddot : Outport
  theta_dot : Outport  Port=2
  theta : Outport  Port=3
  wires:
  Integrator1/1 -> theta/1
  Integrator/1 -> theta_dot/1, Integrator1/1
  Add/1 -> Gain/1
  F_FL/1 -> Add/1
  F_FR/1 -> Add/2
  Add1/1 -> Gain1/1
  F_RR/1 -> Add1/2
  F_RL/1 -> Add1/1
  Gain/1 -> Add2/1
  Gain1/1 -> Add2/2
  Add2/1 -> Gain2/1
  Gain2/1 -> Integrator/1, theta_ddot/1

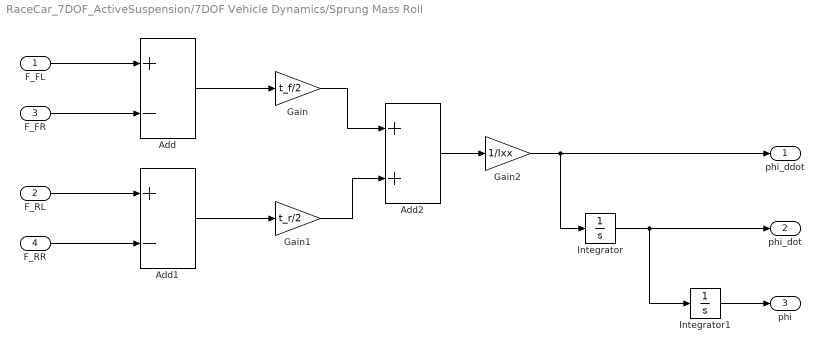
== system RaceCar_7DOF_ActiveSuspension/7DOF Vehicle Dynamics/Sprung Mass Roll ==
  F_FL : Inport
  F_RL : Inport  Port=2
  F_FR : Inport  Port=3
  F_RR : Inport  Port=4
  Add : Sum  Inputs=+-
  Add1 : Sum  Inputs=+-
  Add2 : Sum
  Gain : Gain  Gain=t_f/2
  Gain1 : Gain  Gain=t_r/2
  Gain2 : Gain  Gain=1/Ixx
  Integrator : Integrator  InitialCondition=phi_dot0
  Integrator1 : Integrator  InitialCondition=phi0
  phi_ddot : Outport
  phi_dot : Outport  Port=2
  phi : Outport  Port=3
  wires:
  Gain2/1 -> phi_ddot/1, Integrator/1
  Add2/1 -> Gain2/1
  Gain1/1 -> Add2/2
  Gain/1 -> Add2/1
  F_RL/1 -> Add1/1
  F_RR/1 -> Add1/2
  Add1/1 -> Gain1/1
  F_FR/1 -> Add/2
  F_FL/1 -> Add/1
  Add/1 -> Gain/1
  Integrator/1 -> Integrator1/1, phi_dot/1
  Integrator1/1 -> phi/1

== matlab function RaceCar_7DOF_ActiveSuspension/Asymmetric Kerb Input ==
  data: t input; z_r_FL output; kerb_height input; kerb_duration input; t_kerb_front input; t_kerb_rear input; z_r_FR output; z_r_RL output; z_r_RR output
function [z_r_FL, z_r_FR, z_r_RL, z_r_RR] = ...
    kerb_input(t, kerb_height, kerb_duration, ...
    t_kerb_front, t_kerb_rear)

% Default road heights
z_r_FL = 0;
z_r_FR = 0;
z_r_RL = 0;
z_r_RR = 0;

%% Front-left kerb

if t >= t_kerb_front && ...
   t <= (t_kerb_front + kerb_duration)

    tau = t - t_kerb_front;

    z_r_FL = (kerb_height/2) * ...
        (1 - cos(2*pi*tau/kerb_duration));

end


%% Rear-left kerb

if t >= t_kerb_rear && ...
   t <= (t_kerb_rear + kerb_duration)

    tau = t - t_kerb_rear;

    z_r_RL = (kerb_height/2) * ...
        (1 - cos(2*pi*tau/kerb_duration));

end

end

== matlab function RaceCar_7DOF_ActiveSuspension/Symmetric bump ==
  data: t input; z_r_FL output; bump_height input; bump_duration input; t_bump_front input; t_bump_rear input; z_r_FR output; z_r_RL output; z_r_RR output
function [z_r_FL, z_r_FR, z_r_RL, z_r_RR] = ...
    bump_input(t, bump_height, bump_duration, ...
    t_bump_front, t_bump_rear)

% Default road height
z_r_FL = 0;
z_r_FR = 0;
z_r_RL = 0;
z_r_RR = 0;

%% Front axle bump

if t >= t_bump_front && ...
   t <= (t_bump_front + bump_duration)

    tau = t - t_bump_front;

    z_front = (bump_height/2) * ...
        (1 - cos(2*pi*tau/bump_duration));

    z_r_FL = z_front;
    z_r_FR = z_front;
end


%% Rear axle bump

if t >= t_bump_rear && ...
   t <= (t_bump_rear + bump_duration)

    tau = t - t_bump_rear;

    z_rear = (bump_height/2) * ...
        (1 - cos(2*pi*tau/bump_duration));

    z_r_RL = z_rear;
    z_r_RR = z_rear;
end

end
